simulink model "RC_top_ACU"  (R2018b)
settings: Solver=VariableStepAuto  StartTime=0.0  StopTime=500000.0  RelTol=1e-3
libraries: simulink x4
(part 2 of 3)

== system RC_top_ACU/Global Model RC/ACU/C_steam_4 ==
  from_T_prev_point : Inport
  from_T_curr_point : Inport  Port=2
  init_condition_curr_point : Inport  Port=3
  EVAP_params : Inport  Port=4
  from_prev_point : Inport  Port=5
  from_liquid : Inport  Port=6
  C_steam : Integrator  InitialConditionSource=external  InitialCondition=156.9966
  Gain29 : Gain  Gain=0.0000216487318*10^(-9)
  Sum3 : Sum  Inputs=-+-
  k1 : Subsystem
  speed : Subsystem
  to_next_point : Outport
  to_liquid : Outport  Port=2
  wires:
  init_condition_curr_point/1 -> C_steam/2
  speed/1(Out1) -> Sum3/2
  Gain29/1 -> Sum3/3
  Sum3/1 -> C_steam/1
  from_liquid/1 -> Gain29/1
  k1/1(Out1) -> Sum3/1
  C_steam/1 -> k1/2(In2), to_next_point/1, to_liquid/1
  from_T_curr_point/1 -> k1/1(In1)
  EVAP_params/1 -> k1/3(EVAP_params1), speed/3(EVAP_params)
  from_prev_point/1 -> speed/1(In1)
  from_T_prev_point/1 -> speed/2(In2)

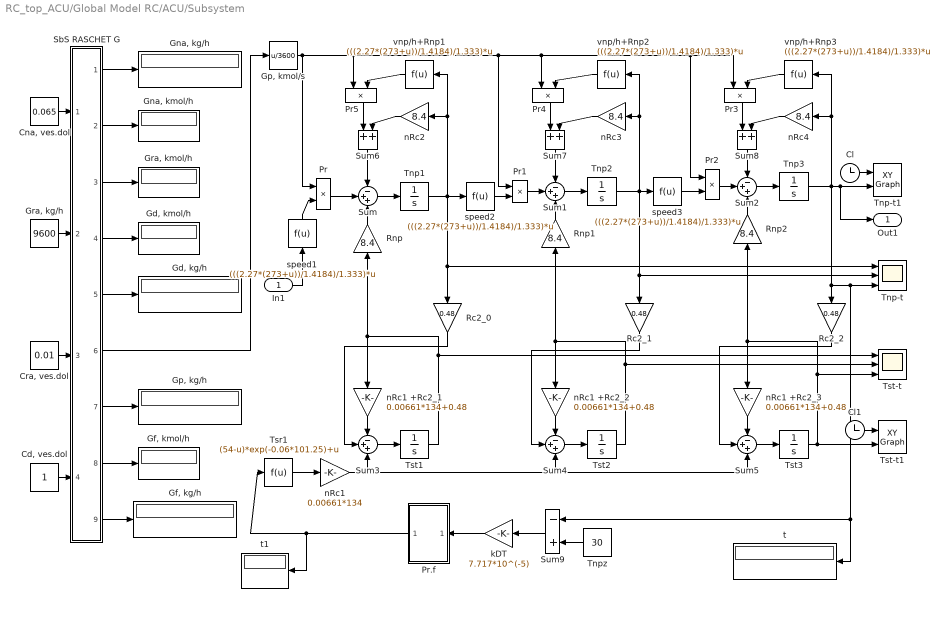
== system RC_top_ACU/Global Model RC/ACU/Subsystem ==
  In1 : Inport
  "Cd, ves.dol" : Constant
  Cl : Clock
  Cl1 : Clock
  "Cna, ves.dol" : Constant  Value=0.065
  "Cra, ves.dol" : Constant  Value=0.01
  "Gd, kg/h" : Display
  "Gd, kmol/h" : Display
  "Gf, kg/h" : Display
  "Gf, kmol/h" : Display
  "Gna, kg/h" : Display
  "Gna, kmol/h" : Display
  "Gp, kmol/s" : Fcn  Expr=u/3600
  "Gp, kg/h" : Display
  "Gra, kg/h" : Constant  Value=9600
  "Gra, kmol/h" : Display
  Pr{,1..5} (6 alike) : Product  RndMeth=Zero
  Pr.f : Subsystem
  Rc2_0 : Gain  Gain=0.48
  Rc2_1 : Gain  Gain=0.48
  Rc2_2 : Gain  Gain=0.48
  Rnp : Gain  Gain=8.4
  Rnp1 : Gain  Gain=8.4
  Rnp2 : Gain  Gain=8.4
  SbS RASCHET G : Subsystem
  Sum{,1..5} (6 alike) : Sum  Inputs=-++
  Sum6 : Sum
  Sum7 : Sum
  Sum8 : Sum
  Sum9 : Sum  Inputs=-+
  Tnp-t : Scope  NumInputPorts=3
  Tnp-t1 : simulink/Sinks/XY Graph  xmin=0  xmax=1000  ymin=10  ymax=50  st=-1
  Tnp1 : Integrator  InitialCondition=55.042986606641151
  Tnp2 : Integrator  InitialCondition=42.494060413287038
  Tnp3 : Integrator  InitialCondition=33.818616670435347
  Tnpz : Constant  Value=30
  Tsr1 : Fcn  Expr=(54-u)*exp(-0.06*101.25)+u
  Tst-t : Scope  NumInputPorts=3
  Tst-t1 : simulink/Sinks/XY Graph  xmin=0  xmax=1000  ymin=10  ymax=50  st=-1
  Tst1 : Integrator  InitialCondition=30.749212884999000
  Tst2 : Integrator  InitialCondition=26.338794670104530
  Tst3 : Integrator  InitialCondition=23.289742144317184
  kDT : Gain  Gain=7.717*10^(-5)
  nRc1 : Gain  Gain=0.00661*134
  nRc1 +Rc2_1 : Gain  Gain=0.00661*134+0.48
  nRc1 +Rc2_2 : Gain  Gain=0.00661*134+0.48
  nRc1 +Rc2_3 : Gain  Gain=0.00661*134+0.48
  nRc2 : Gain  Gain=8.4
  nRc3 : Gain  Gain=8.4
  nRc4 : Gain  Gain=8.4
  speed1 : Fcn  Expr=(((2.27*(273+u))/1.4184)/1.333)*u
  speed2 : Fcn  Expr=(((2.27*(273+u))/1.4184)/1.333)*u
  speed3 : Fcn  Expr=(((2.27*(273+u))/1.4184)/1.333)*u
  t : Display
  t1 : Display
  vnp/h+Rnp1 : Fcn  Expr=(((2.27*(273+u))/1.4184)/1.333)*u
  vnp/h+Rnp2 : Fcn  Expr=(((2.27*(273+u))/1.4184)/1.333)*u
  vnp/h+Rnp3 : Fcn  Expr=(((2.27*(273+u))/1.4184)/1.333)*u
  Out1 : Outport
  wires:
  Sum/1 -> Tnp1/1
  Tnp1/1 -> speed2/1, Rc2_0/1, Tnp-t/1, vnp/h+Rnp1/1, nRc2/1
  Sum1/1 -> Tnp2/1
  Tnp2/1 -> speed3/1, Rc2_1/1, Tnp-t/2, vnp/h+Rnp2/1, nRc3/1
  Sum2/1 -> Tnp3/1
  Tnp3/1 -> vnp/h+Rnp3/1, nRc4/1, Tnp-t1/2, Out1/1, Rc2_2/1, Tnp-t/3, t/1, Sum9/1
  Cl/1 -> Tnp-t1/1
  Rnp1/1 -> Sum1/3
  Rnp2/1 -> Sum2/3
  nRc1 +Rc2_1/1 -> Sum3/1
  Sum3/1 -> Tst1/1
  nRc1 +Rc2_2/1 -> Sum4/1
  Sum4/1 -> Tst2/1
  Tst2/1 -> nRc1 +Rc2_2/1, Rnp1/1, Tst-t/2
  nRc1 +Rc2_3/1 -> Sum5/1
  Sum5/1 -> Tst3/1
  nRc1/1 -> Sum3/3, Sum5/3, Sum4/3
  Rnp/1 -> Sum/3
  Tst1/1 -> nRc1 +Rc2_1/1, Rnp/1, Tst-t/1
  Tst3/1 -> Tst-t1/2, nRc1 +Rc2_3/1, Rnp2/1, Tst-t/3
  Rc2_1/1 -> Sum4/2
  Rc2_2/1 -> Sum5/2
  Rc2_0/1 -> Sum3/2
  Cl1/1 -> Tst-t1/1
  speed1/1 -> Pr/2
  "Gp, kmol/s"/1 -> Pr/1, Pr5/1, Pr2/1, Pr3/1, Pr4/1, Pr1/1
  Pr/1 -> Sum/2
  Pr1/1 -> Sum1/2
  speed2/1 -> Pr1/2
  Pr2/1 -> Sum2/2
  speed3/1 -> Pr2/2
  vnp/h+Rnp3/1 -> Pr3/2
  vnp/h+Rnp2/1 -> Pr4/2
  vnp/h+Rnp1/1 -> Pr5/2
  Pr5/1 -> Sum6/1
  Sum6/1 -> Sum/1
  nRc2/1 -> Sum6/2
  nRc3/1 -> Sum7/2
  Pr4/1 -> Sum7/1
  Sum7/1 -> Sum1/1
  nRc4/1 -> Sum8/2
  Pr3/1 -> Sum8/1
  Sum8/1 -> Sum2/1
  "Cna, ves.dol"/1 -> SbS RASCHET G/1(In1)
  "Cra, ves.dol"/1 -> SbS RASCHET G/3(In3)
  "Cd, ves.dol"/1 -> SbS RASCHET G/4(In4)
  "Gra, kg/h"/1 -> SbS RASCHET G/2(In2)
  SbS RASCHET G/1(Out1) -> "Gna, kg/h"/1
  SbS RASCHET G/5(Out5) -> "Gd, kg/h"/1
  SbS RASCHET G/7(Out7) -> "Gp, kg/h"/1
  SbS RASCHET G/9(Out9) -> "Gf, kg/h"/1
  SbS RASCHET G/2(Out2) -> "Gna, kmol/h"/1
  SbS RASCHET G/3(Out3) -> "Gra, kmol/h"/1
  SbS RASCHET G/4(Out4) -> "Gd, kmol/h"/1
  SbS RASCHET G/6(Out6) -> "Gp, kmol/s"/1
  SbS RASCHET G/8(Out8) -> "Gf, kmol/h"/1
  In1/1 -> speed1/1
  Sum9/1 -> kDT/1
  Tnpz/1 -> Sum9/2
  Pr.f/1(Out1) -> t1/1, Tsr1/1
  kDT/1 -> Pr.f/1(In1)
  Tsr1/1 -> nRc1/1

== system RC_top_ACU/Global Model RC/ACU/T_flue_1 ==
  init_condition_curr_point : Inport
  from_prev_point : Inport  Port=2
  from_side : Inport  Port=3
  Rdg : Gain  Gain=0.47
  Sum2 : Sum  Inputs=++-
  T_flue : Integrator  InitialConditionSource=external  InitialCondition=124.3766
  Vdg/h : Gain  Gain=4.6/1.375
  vdg/h+Rdg : Gain  Gain=4.6/1.375+0.47
  to_next_point : Outport
  to_side : Outport  Port=2
  wires:
  Vdg/h/1 -> Sum2/2
  from_prev_point/1 -> Vdg/h/1
  from_side/1 -> Rdg/1
  vdg/h+Rdg/1 -> Sum2/3
  Sum2/1 -> T_flue/1
  Rdg/1 -> Sum2/1
  init_condition_curr_point/1 -> T_flue/2
  T_flue/1 -> to_next_point/1, vdg/h+Rdg/1, to_side/1

== system RC_top_ACU/Global Model RC/ACU/T_flue_2 ==
  init_condition_curr_point : Inport
  from_prev_point : Inport  Port=2
  from_side : Inport  Port=3
  Rdg : Gain  Gain=0.47
  Sum2 : Sum  Inputs=++-
  T_flue : Integrator  InitialConditionSource=external  InitialCondition=124.3766
  Vdg/h : Gain  Gain=4.6/1.375
  vdg/h+Rdg : Gain  Gain=4.6/1.375+0.47
  to_next_point : Outport
  to_side : Outport  Port=2
  wires:
  Vdg/h/1 -> Sum2/2
  from_prev_point/1 -> Vdg/h/1
  from_side/1 -> Rdg/1
  vdg/h+Rdg/1 -> Sum2/3
  Sum2/1 -> T_flue/1
  Rdg/1 -> Sum2/1
  init_condition_curr_point/1 -> T_flue/2
  T_flue/1 -> to_next_point/1, vdg/h+Rdg/1, to_side/1

== system RC_top_ACU/Global Model RC/ACU/T_flue_3 ==
  init_condition_curr_point : Inport
  from_prev_point : Inport  Port=2
  from_side : Inport  Port=3
  Rdg : Gain  Gain=0.47
  Sum2 : Sum  Inputs=++-
  T_flue : Integrator  InitialConditionSource=external  InitialCondition=124.3766
  Vdg/h : Gain  Gain=4.6/1.375
  vdg/h+Rdg : Gain  Gain=4.6/1.375+0.47
  to_next_point : Outport
  to_side : Outport  Port=2
  wires:
  Vdg/h/1 -> Sum2/2
  from_prev_point/1 -> Vdg/h/1
  from_side/1 -> Rdg/1
  vdg/h+Rdg/1 -> Sum2/3
  Sum2/1 -> T_flue/1
  Rdg/1 -> Sum2/1
  init_condition_curr_point/1 -> T_flue/2
  T_flue/1 -> to_next_point/1, vdg/h+Rdg/1, to_side/1

== system RC_top_ACU/Global Model RC/ACU/T_flue_4 ==
  init_condition_curr_point : Inport
  from_prev_point : Inport  Port=2
  from_side : Inport  Port=3
  Rdg : Gain  Gain=0.47
  Sum2 : Sum  Inputs=++-
  T_flue : Integrator  InitialConditionSource=external  InitialCondition=124.3766
  Vdg/h : Gain  Gain=4.6/1.375
  vdg/h+Rdg : Gain  Gain=4.6/1.375+0.47
  to_next_point : Outport
  to_side : Outport  Port=2
  wires:
  Vdg/h/1 -> Sum2/2
  from_prev_point/1 -> Vdg/h/1
  from_side/1 -> Rdg/1
  vdg/h+Rdg/1 -> Sum2/3
  Sum2/1 -> T_flue/1
  Rdg/1 -> Sum2/1
  init_condition_curr_point/1 -> T_flue/2
  T_flue/1 -> to_next_point/1, vdg/h+Rdg/1, to_side/1

== system RC_top_ACU/Global Model RC/ACU/T_liquide_1 ==
  from_side : Inport
  init_condition_curr_point : Inport  Port=2
  from_prev_point : Inport  Port=3
  Ra : Gain  Gain=0.003
  Sum37 : Sum  Inputs=++-
  T_liquide : Integrator  InitialConditionSource=external  InitialCondition=136.285
  va/h+Ra : Gain  Gain=0.003/1.375+0.003
  va/h1 : Gain  Gain=0.003/1.375
  to_side : Outport
  to_next_point : Outport  Port=2
  wires:
  init_condition_curr_point/1 -> T_liquide/2
  va/h1/1 -> Sum37/2
  Sum37/1 -> T_liquide/1
  from_prev_point/1 -> va/h1/1
  Ra/1 -> Sum37/1
  from_side/1 -> Ra/1
  T_liquide/1 -> to_next_point/1, va/h+Ra/1, to_side/1
  va/h+Ra/1 -> Sum37/3

== system RC_top_ACU/Global Model RC/ACU/T_liquide_2 ==
  from_side : Inport
  init_condition_curr_point : Inport  Port=2
  from_prev_point : Inport  Port=3
  Ra : Gain  Gain=0.003
  Sum37 : Sum  Inputs=++-
  T_liquide : Integrator  InitialConditionSource=external  InitialCondition=136.285
  va/h+Ra : Gain  Gain=0.003/1.375+0.003
  va/h1 : Gain  Gain=0.003/1.375
  to_side : Outport
  to_next_point : Outport  Port=2
  wires:
  init_condition_curr_point/1 -> T_liquide/2
  va/h1/1 -> Sum37/2
  Sum37/1 -> T_liquide/1
  from_prev_point/1 -> va/h1/1
  Ra/1 -> Sum37/1
  from_side/1 -> Ra/1
  T_liquide/1 -> to_next_point/1, va/h+Ra/1, to_side/1
  va/h+Ra/1 -> Sum37/3

== system RC_top_ACU/Global Model RC/ACU/T_liquide_3 ==
  from_side : Inport
  init_condition_curr_point : Inport  Port=2
  from_prev_point : Inport  Port=3
  Ra : Gain  Gain=0.003
  Sum37 : Sum  Inputs=++-
  T_liquide : Integrator  InitialConditionSource=external  InitialCondition=136.285
  va/h+Ra : Gain  Gain=0.003/1.375+0.003
  va/h1 : Gain  Gain=0.003/1.375
  to_side : Outport
  to_next_point : Outport  Port=2
  wires:
  init_condition_curr_point/1 -> T_liquide/2
  va/h1/1 -> Sum37/2
  Sum37/1 -> T_liquide/1
  from_prev_point/1 -> va/h1/1
  Ra/1 -> Sum37/1
  from_side/1 -> Ra/1
  T_liquide/1 -> to_next_point/1, va/h+Ra/1, to_side/1
  va/h+Ra/1 -> Sum37/3

== system RC_top_ACU/Global Model RC/ACU/T_liquide_4 ==
  from_side : Inport
  init_condition_curr_point : Inport  Port=2
  from_prev_point : Inport  Port=3
  Ra : Gain  Gain=0.003
  Sum37 : Sum  Inputs=++-
  T_liquide : Integrator  InitialConditionSource=external  InitialCondition=136.285
  va/h+Ra : Gain  Gain=0.003/1.375+0.003
  va/h1 : Gain  Gain=0.003/1.375
  to_side : Outport
  to_next_point : Outport  Port=2
  wires:
  init_condition_curr_point/1 -> T_liquide/2
  va/h1/1 -> Sum37/2
  Sum37/1 -> T_liquide/1
  from_prev_point/1 -> va/h1/1
  Ra/1 -> Sum37/1
  from_side/1 -> Ra/1
  T_liquide/1 -> to_next_point/1, va/h+Ra/1, to_side/1
  va/h+Ra/1 -> Sum37/3

== system RC_top_ACU/Global Model RC/ACU/T_side_1 ==
  from_flue : Inport
  init_condition_curr_point : Inport  Port=2
  from_liquide : Inport  Port=3
  Rast : Gain  Gain=0.22
  Rdgst : Gain  Gain=0.008
  Rdgst+Rast : Gain  Gain=0.008+0.22
  Sum2 : Sum  Inputs=++-
  T_side : Integrator  InitialConditionSource=external  InitialCondition=124.3766
  to_flue : Outport
  to_liquide : Outport  Port=2
  wires:
  Rast/1 -> Sum2/2
  from_liquide/1 -> Rast/1
  from_flue/1 -> Rdgst/1
  T_side/1 -> Rdgst+Rast/1, to_liquide/1, to_flue/1
  Rdgst+Rast/1 -> Sum2/3
  Sum2/1 -> T_side/1
  Rdgst/1 -> Sum2/1
  init_condition_curr_point/1 -> T_side/2

== system RC_top_ACU/Global Model RC/ACU/T_side_2 ==
  from_flue : Inport
  init_condition_curr_point : Inport  Port=2
  from_liquide : Inport  Port=3
  Rast : Gain  Gain=0.22
  Rdgst : Gain  Gain=0.008
  Rdgst+Rast : Gain  Gain=0.008+0.22
  Sum2 : Sum  Inputs=++-
  T_side : Integrator  InitialConditionSource=external  InitialCondition=124.3766
  to_flue : Outport
  to_liquide : Outport  Port=2
  wires:
  Rast/1 -> Sum2/2
  from_liquide/1 -> Rast/1
  from_flue/1 -> Rdgst/1
  T_side/1 -> Rdgst+Rast/1, to_liquide/1, to_flue/1
  Rdgst+Rast/1 -> Sum2/3
  Sum2/1 -> T_side/1
  Rdgst/1 -> Sum2/1
  init_condition_curr_point/1 -> T_side/2

== system RC_top_ACU/Global Model RC/ACU/T_side_3 ==
  from_flue : Inport
  init_condition_curr_point : Inport  Port=2
  from_liquide : Inport  Port=3
  Rast : Gain  Gain=0.22
  Rdgst : Gain  Gain=0.008
  Rdgst+Rast : Gain  Gain=0.008+0.22
  Sum2 : Sum  Inputs=++-
  T_side : Integrator  InitialConditionSource=external  InitialCondition=124.3766
  to_flue : Outport
  to_liquide : Outport  Port=2
  wires:
  Rast/1 -> Sum2/2
  from_liquide/1 -> Rast/1
  from_flue/1 -> Rdgst/1
  T_side/1 -> Rdgst+Rast/1, to_liquide/1, to_flue/1
  Rdgst+Rast/1 -> Sum2/3
  Sum2/1 -> T_side/1
  Rdgst/1 -> Sum2/1
  init_condition_curr_point/1 -> T_side/2

== system RC_top_ACU/Global Model RC/ACU/T_side_4 ==
  from_flue : Inport
  init_condition_curr_point : Inport  Port=2
  from_liquide : Inport  Port=3
  Rast : Gain  Gain=0.22
  Rdgst : Gain  Gain=0.008
  Rdgst+Rast : Gain  Gain=0.008+0.22
  Sum2 : Sum  Inputs=++-
  T_side : Integrator  InitialConditionSource=external  InitialCondition=124.3766
  to_flue : Outport
  to_liquide : Outport  Port=2
  wires:
  Rast/1 -> Sum2/2
  from_liquide/1 -> Rast/1
  from_flue/1 -> Rdgst/1
  T_side/1 -> Rdgst+Rast/1, to_liquide/1, to_flue/1
  Rdgst+Rast/1 -> Sum2/3
  Sum2/1 -> T_side/1
  Rdgst/1 -> Sum2/1
  init_condition_curr_point/1 -> T_side/2

== system RC_top_ACU/Global Model RC/ACU/T_steam ==
  point_1 : Inport
  point_3 : Inport  Port=2
  point_2 : Inport  Port=3
  point_4 : Inport  Port=4
  Gain : Gain  Gain=1/4
  Sum37 : Sum  Inputs=++++
  to_side : Outport
  wires:
  point_2/1 -> Sum37/2
  point_1/1 -> Sum37/1
  point_3/1 -> Sum37/3
  point_4/1 -> Sum37/4
  Sum37/1 -> Gain/1
  Gain/1 -> to_side/1

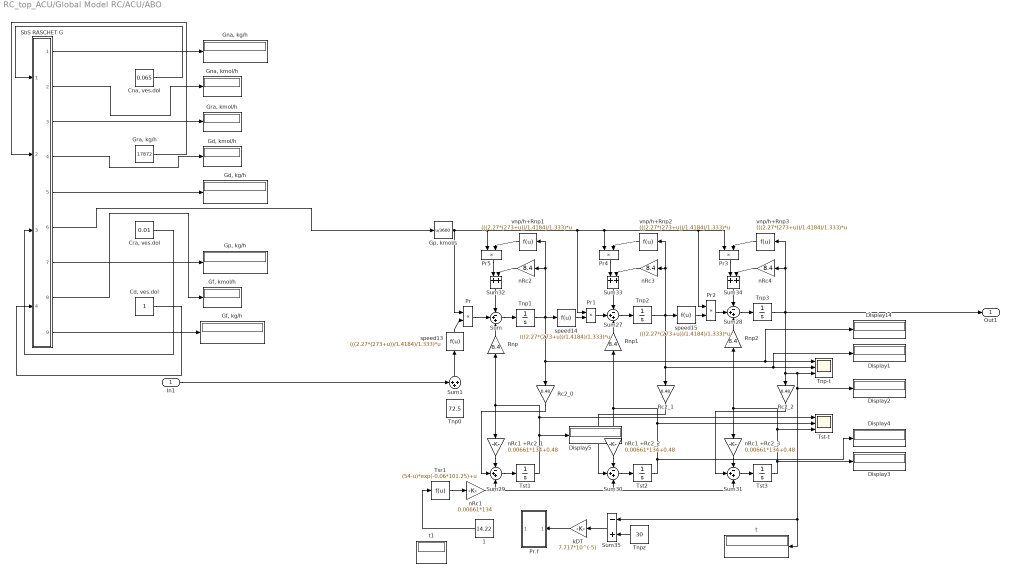
== system RC_top_ACU/Global Model RC/ACU/АВО ==
  In1 : Inport
  1 : Constant  Value=14.22
  "Cd, ves.dol" : Constant
  "Cna, ves.dol" : Constant  Value=0.065
  "Cra, ves.dol" : Constant  Value=0.01
  Display{1..5,14} (6 alike) : Display
  "Gd, kg/h" : Display
  "Gd, kmol/h" : Display
  "Gf, kg/h" : Display
  "Gf, kmol/h" : Display
  "Gna, kg/h" : Display
  "Gna, kmol/h" : Display
  "Gp, kmol/s" : Fcn  Expr=u/3600
  "Gp, kg/h" : Display
  "Gra, kg/h" : Constant  Value=17872
  "Gra, kmol/h" : Display
  Pr{,1..5} (6 alike) : Product  RndMeth=Zero
  Pr.f : Subsystem
  Rc2_0 : Gain  Gain=0.48
  Rc2_1 : Gain  Gain=0.48
  Rc2_2 : Gain  Gain=0.48
  Rnp : Gain  Gain=8.4
  Rnp1 : Gain  Gain=8.4
  Rnp2 : Gain  Gain=8.4
  SbS RASCHET G : Subsystem
  Sum{,27..31} (6 alike) : Sum  Inputs=-++
  Sum1 : Sum  Inputs=+++
  Sum32 : Sum
  Sum33 : Sum
  Sum34 : Sum
  Sum35 : Sum  Inputs=-+
  Tnp-t : Scope  NumInputPorts=3
  Tnp0 : Constant  Value=72.5
  Tnp1 : Integrator  InitialCondition=64.9985
  Tnp2 : Integrator  InitialCondition=57.497
  Tnp3 : Integrator  InitialCondition=49.9955
  Tnpz : Constant  Value=30
  Tsr1 : Fcn  Expr=(54-u)*exp(-0.06*101.25)+u
  Tst-t : Scope  NumInputPorts=3
  Tst1 : Integrator  InitialCondition=30.75
  Tst2 : Integrator  InitialCondition=27.02
  Tst3 : Integrator  InitialCondition=23.29
  kDT : Gain  Gain=7.717*10^(-5)
  nRc1 : Gain  Gain=0.00661*134
  nRc1 +Rc2_1 : Gain  Gain=0.00661*134+0.48
  nRc1 +Rc2_2 : Gain  Gain=0.00661*134+0.48
  nRc1 +Rc2_3 : Gain  Gain=0.00661*134+0.48
  nRc2 : Gain  Gain=8.4
  nRc3 : Gain  Gain=8.4
  nRc4 : Gain  Gain=8.4
  speed13 : Fcn  Expr=(((2.27*(273+u))/1.4184)/1.333)*u
  speed14 : Fcn  Expr=(((2.27*(273+u))/1.4184)/1.333)*u
  speed15 : Fcn  Expr=(((2.27*(273+u))/1.4184)/1.333)*u
  t : Display
  t1 : Display
  vnp/h+Rnp1 : Fcn  Expr=(((2.27*(273+u))/1.4184)/1.333)*u
  vnp/h+Rnp2 : Fcn  Expr=(((2.27*(273+u))/1.4184)/1.333)*u
  vnp/h+Rnp3 : Fcn  Expr=(((2.27*(273+u))/1.4184)/1.333)*u
  Out1 : Outport
  wires:
  Sum/1 -> Tnp1/1
  Tnp2/1 -> speed15/1, Rc2_1/1, Display1/1, Tnp-t/2, vnp/h+Rnp2/1, nRc3/1
  Tnp1/1 -> speed14/1, Rc2_0/1, Display14/1, Tnp-t/1, vnp/h+Rnp1/1, nRc2/1
  Sum27/1 -> Tnp2/1
  Sum28/1 -> Tnp3/1
  vnp/h+Rnp3/1 -> Pr3/2
  vnp/h+Rnp2/1 -> Pr4/2
  vnp/h+Rnp1/1 -> Pr5/2
  Sum32/1 -> Sum/1
  Rnp2/1 -> Sum28/3
  Pr4/1 -> Sum33/1
  "Cra, ves.dol"/1 -> SbS RASCHET G/3(In3)
  Sum31/1 -> Tst3/1
  "Cd, ves.dol"/1 -> SbS RASCHET G/4(In4)
  nRc1 +Rc2_1/1 -> Sum29/1
  Tst1/1 -> Display5/1, nRc1 +Rc2_1/1, Rnp/1, Tst-t/1
  "Gra, kg/h"/1 -> SbS RASCHET G/2(In2)
  SbS RASCHET G/1(Out1) -> "Gna, kg/h"/1
  SbS RASCHET G/5(Out5) -> "Gd, kg/h"/1
  Sum29/1 -> Tst1/1
  Pr/1 -> Sum/2
  Rc2_2/1 -> Sum31/2
  speed14/1 -> Pr1/2
  Rnp/1 -> Sum/3
  nRc1/1 -> Sum29/3, Sum31/3, Sum30/3
  "Gp, kmol/s"/1 -> Pr/1, Pr5/1, Pr2/1, Pr3/1, Pr4/1, Pr1/1
  Tnp3/1 -> vnp/h+Rnp3/1, nRc4/1, Out1/1, Rc2_2/1, Tnp-t/3, Display2/1, t/1, Sum35/1
  Tst3/1 -> Display3/1, nRc1 +Rc2_3/1, Rnp2/1, Tst-t/3
  Sum30/1 -> Tst2/1
  Pr5/1 -> Sum32/1
  Rc2_1/1 -> Sum30/2
  nRc1 +Rc2_3/1 -> Sum31/1
  Pr2/1 -> Sum28/2
  nRc2/1 -> Sum32/2
  nRc3/1 -> Sum33/2
  "Cna, ves.dol"/1 -> SbS RASCHET G/1(In1)
  speed15/1 -> Pr2/2
  Sum33/1 -> Sum27/1
  nRc4/1 -> Sum34/2
  Sum34/1 -> Sum28/1
  nRc1 +Rc2_2/1 -> Sum30/1
  Rnp1/1 -> Sum27/3
  Pr1/1 -> Sum27/2
  Pr3/1 -> Sum34/1
  speed13/1 -> Pr/2
  Tst2/1 -> nRc1 +Rc2_2/1, Rnp1/1, Tst-t/2, Display4/1
  Rc2_0/1 -> Sum29/2
  SbS RASCHET G/7(Out7) -> "Gp, kg/h"/1
  SbS RASCHET G/6(Out6) -> "Gp, kmol/s"/1
  SbS RASCHET G/4(Out4) -> "Gd, kmol/h"/1
  Tsr1/1 -> nRc1/1
  SbS RASCHET G/2(Out2) -> "Gna, kmol/h"/1
  SbS RASCHET G/3(Out3) -> "Gra, kmol/h"/1
  SbS RASCHET G/9(Out9) -> "Gf, kg/h"/1
  Sum35/1 -> kDT/1
  Tnpz/1 -> Sum35/2
  kDT/1 -> Pr.f/1(In1)
  SbS RASCHET G/8(Out8) -> "Gf, kmol/h"/1
  Sum1/1 -> speed13/1
  In1/1 -> Sum1/1
  1/1 -> Tsr1/1

== system RC_top_ACU/Global Model RC/FULL_RC_1/k19 ==
  In1 : Inport
  In2 : Inport  Port=2
  Product13 : Product  SaturateOnIntegerOverflow=on  InputSameDT=on  OutDataTypeStr=Inherit: Same as first input
  speed3 : Fcn  Expr=(0.002702752*(273.15+u))/1.17-0.147
  Out1 : Outport
  wires:
  Product13/1 -> Out1/1
  speed3/1 -> Product13/2
  In2/1 -> speed3/1
  In1/1 -> Product13/1

== system RC_top_ACU/Global Model RC/FULL_RC_1/k23 ==
  In1 : Inport
  In2 : Inport  Port=2
  Product13 : Product  SaturateOnIntegerOverflow=on  InputSameDT=on  OutDataTypeStr=Inherit: Same as first input
  speed3 : Fcn  Expr=(0.002702752*(273.15+u))/1.17-0.147
  Out1 : Outport
  wires:
  In1/1 -> Product13/1
  In2/1 -> speed3/1
  speed3/1 -> Product13/2
  Product13/1 -> Out1/1

== system RC_top_ACU/Global Model RC/FULL_RC_1/k24 ==
  In1 : Inport
  In2 : Inport  Port=2
  Product13 : Product  SaturateOnIntegerOverflow=on  InputSameDT=on  OutDataTypeStr=Inherit: Same as first input
  speed3 : Fcn  Expr=(0.002702752*(273.15+u))/1.17-0.147
  Out1 : Outport
  wires:
  Product13/1 -> Out1/1
  speed3/1 -> Product13/2
  In2/1 -> speed3/1
  In1/1 -> Product13/1

== system RC_top_ACU/Global Model RC/FULL_RC_1/k28 ==
  In1 : Inport
  In2 : Inport  Port=2
  Product13 : Product  SaturateOnIntegerOverflow=on  InputSameDT=on  OutDataTypeStr=Inherit: Same as first input
  speed3 : Fcn  Expr=((0.003223135*(273+u))/24.69822264)/0.5-0.004302
  Out1 : Outport
  wires:
  Product13/1 -> Out1/1
  speed3/1 -> Product13/1
  In1/1 -> speed3/1
  In2/1 -> Product13/2

== system RC_top_ACU/Global Model RC/FULL_RC_1/k29 ==
  In1 : Inport
  In2 : Inport  Port=2
  Product13 : Product  SaturateOnIntegerOverflow=on  InputSameDT=on  OutDataTypeStr=Inherit: Same as first input
  speed3 : Fcn  Expr=((0.003223135*(273+u))/24.69822264)/0.5-0.004302
  Out1 : Outport
  wires:
  Product13/1 -> Out1/1
  speed3/1 -> Product13/1
  In1/1 -> speed3/1
  In2/1 -> Product13/2

== system RC_top_ACU/Global Model RC/FULL_RC_1/k30 ==
  In1 : Inport
  In2 : Inport  Port=2
  Product13 : Product  SaturateOnIntegerOverflow=on  InputSameDT=on  OutDataTypeStr=Inherit: Same as first input
  speed3 : Fcn  Expr=((0.003223135*(273+u))/24.69822264)/0.5-0.004302
  Out1 : Outport
  wires:
  Product13/1 -> Out1/1
  speed3/1 -> Product13/1
  In1/1 -> speed3/1
  In2/1 -> Product13/2

== system RC_top_ACU/Global Model RC/FULL_RC_1/speed22 ==
  In1 : Inport
  In2 : Inport  Port=2
  Product13 : Product  SaturateOnIntegerOverflow=on  InputSameDT=on  OutDataTypeStr=Inherit: Same as first input
  speed3 : Fcn  Expr=(0.002702752*(273.15+u))/1.17
  Out1 : Outport
  wires:
  Product13/1 -> Out1/1
  speed3/1 -> Product13/2
  In2/1 -> speed3/1
  In1/1 -> Product13/1

== system RC_top_ACU/Global Model RC/FULL_RC_1/speed25 ==
  In1 : Inport
  In2 : Inport  Port=2
  Product13 : Product  SaturateOnIntegerOverflow=on  InputSameDT=on  OutDataTypeStr=Inherit: Same as first input
  speed3 : Fcn  Expr=((0.003223135*(273+u))/24.69822264)/0.5
  Out1 : Outport
  wires:
  In1/1 -> Product13/1
  In2/1 -> speed3/1
  speed3/1 -> Product13/2
  Product13/1 -> Out1/1

== system RC_top_ACU/Global Model RC/FULL_RC_1/speed26 ==
  In1 : Inport
  In2 : Inport  Port=2
  Product13 : Product  SaturateOnIntegerOverflow=on  InputSameDT=on  OutDataTypeStr=Inherit: Same as first input
  speed3 : Fcn  Expr=(0.002702752*(273.15+u))/1.17
  Out1 : Outport
  wires:
  In1/1 -> Product13/1
  In2/1 -> speed3/1
  speed3/1 -> Product13/2
  Product13/1 -> Out1/1

== system RC_top_ACU/Global Model RC/FULL_RC_1/speed30 ==
  In1 : Inport
  In2 : Inport  Port=2
  Product13 : Product  SaturateOnIntegerOverflow=on  InputSameDT=on  OutDataTypeStr=Inherit: Same as first input
  speed3 : Fcn  Expr=(0.002702752*(273.15+u))/1.17
  Out1 : Outport
  wires:
  In1/1 -> Product13/1
  In2/1 -> speed3/1
  speed3/1 -> Product13/2
  Product13/1 -> Out1/1

== system RC_top_ACU/Global Model RC/FULL_RC_1/speed31 ==
  In1 : Inport
  In2 : Inport  Port=2
  Product13 : Product  SaturateOnIntegerOverflow=on  InputSameDT=on  OutDataTypeStr=Inherit: Same as first input
  speed3 : Fcn  Expr=((0.003223135*(273+u))/24.69822264)/0.5
  Out1 : Outport
  wires:
  Product13/1 -> Out1/1
  In2/1 -> Product13/2
  speed3/1 -> Product13/1
  In1/1 -> speed3/1

== system RC_top_ACU/Global Model RC/FULL_RC_1/speed32 ==
  In1 : Inport
  In2 : Inport  Port=2
  Product13 : Product  SaturateOnIntegerOverflow=on  InputSameDT=on  OutDataTypeStr=Inherit: Same as first input
  speed3 : Fcn  Expr=((0.003223135*(273+u))/24.69822264)/0.5
  Out1 : Outport
  wires:
  Product13/1 -> Out1/1
  In2/1 -> Product13/2
  speed3/1 -> Product13/1
  In1/1 -> speed3/1

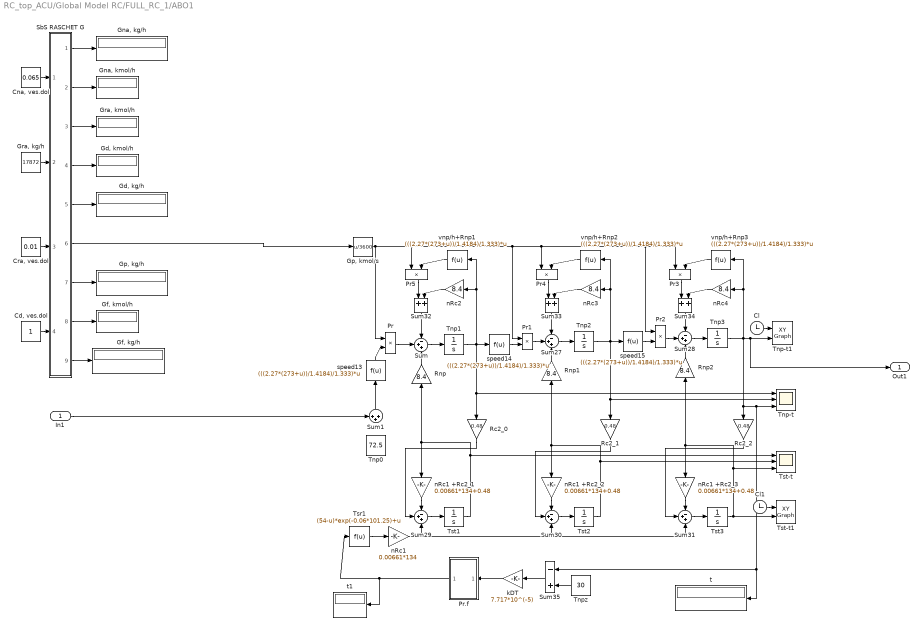
== system RC_top_ACU/Global Model RC/FULL_RC_1/АВО1 ==
  In1 : Inport
  "Cd, ves.dol" : Constant
  Cl : Clock
  Cl1 : Clock
  "Cna, ves.dol" : Constant  Value=0.065
  "Cra, ves.dol" : Constant  Value=0.01
  "Gd, kg/h" : Display
  "Gd, kmol/h" : Display
  "Gf, kg/h" : Display
  "Gf, kmol/h" : Display
  "Gna, kg/h" : Display
  "Gna, kmol/h" : Display
  "Gp, kmol/s" : Fcn  Expr=u/3600
  "Gp, kg/h" : Display
  "Gra, kg/h" : Constant  Value=17872
  "Gra, kmol/h" : Display
  Pr{,1..5} (6 alike) : Product  RndMeth=Zero
  Pr.f : Subsystem
  Rc2_0 : Gain  Gain=0.48
  Rc2_1 : Gain  Gain=0.48
  Rc2_2 : Gain  Gain=0.48
  Rnp : Gain  Gain=8.4
  Rnp1 : Gain  Gain=8.4
  Rnp2 : Gain  Gain=8.4
  SbS RASCHET G : Subsystem
  Sum{,27..31} (6 alike) : Sum  Inputs=-++
  Sum1 : Sum  Inputs=+++
  Sum32 : Sum
  Sum33 : Sum
  Sum34 : Sum
  Sum35 : Sum  Inputs=-+
  Tnp-t : Scope  NumInputPorts=3
  Tnp-t1 : simulink/Sinks/XY Graph  xmin=0  xmax=1000  ymin=10  ymax=50  st=-1
  Tnp0 : Constant  Value=72.5
  Tnp1 : Integrator  InitialCondition=55.042986606641151
  Tnp2 : Integrator  InitialCondition=42.494060413287038
  Tnp3 : Integrator  InitialCondition=33.818616670435347
  Tnpz : Constant  Value=30
  Tsr1 : Fcn  Expr=(54-u)*exp(-0.06*101.25)+u
  Tst-t : Scope  NumInputPorts=3
  Tst-t1 : simulink/Sinks/XY Graph  xmin=0  xmax=1000  ymin=10  ymax=50  st=-1
  Tst1 : Integrator  InitialCondition=30.749212884999000
  Tst2 : Integrator  InitialCondition=26.338794670104530
  Tst3 : Integrator  InitialCondition=23.289742144317184
  kDT : Gain  Gain=7.717*10^(-5)
  nRc1 : Gain  Gain=0.00661*134
  nRc1 +Rc2_1 : Gain  Gain=0.00661*134+0.48
  nRc1 +Rc2_2 : Gain  Gain=0.00661*134+0.48
  nRc1 +Rc2_3 : Gain  Gain=0.00661*134+0.48
  nRc2 : Gain  Gain=8.4
  nRc3 : Gain  Gain=8.4
  nRc4 : Gain  Gain=8.4
  speed13 : Fcn  Expr=(((2.27*(273+u))/1.4184)/1.333)*u
  speed14 : Fcn  Expr=(((2.27*(273+u))/1.4184)/1.333)*u
  speed15 : Fcn  Expr=(((2.27*(273+u))/1.4184)/1.333)*u
  t : Display
  t1 : Display
  vnp/h+Rnp1 : Fcn  Expr=(((2.27*(273+u))/1.4184)/1.333)*u
  vnp/h+Rnp2 : Fcn  Expr=(((2.27*(273+u))/1.4184)/1.333)*u
  vnp/h+Rnp3 : Fcn  Expr=(((2.27*(273+u))/1.4184)/1.333)*u
  Out1 : Outport
  wires:
  Sum/1 -> Tnp1/1
  Tnp2/1 -> speed15/1, Rc2_1/1, Tnp-t/2, vnp/h+Rnp2/1, nRc3/1
  Tnp1/1 -> speed14/1, Rc2_0/1, Tnp-t/1, vnp/h+Rnp1/1, nRc2/1
  Sum27/1 -> Tnp2/1
  Sum28/1 -> Tnp3/1
  vnp/h+Rnp3/1 -> Pr3/2
  vnp/h+Rnp2/1 -> Pr4/2
  vnp/h+Rnp1/1 -> Pr5/2
  Sum32/1 -> Sum/1
  Rnp2/1 -> Sum28/3
  Pr4/1 -> Sum33/1
  "Cra, ves.dol"/1 -> SbS RASCHET G/3(In3)
  Sum31/1 -> Tst3/1
  "Cd, ves.dol"/1 -> SbS RASCHET G/4(In4)
  Cl/1 -> Tnp-t1/1
  nRc1 +Rc2_1/1 -> Sum29/1
  Tst1/1 -> nRc1 +Rc2_1/1, Rnp/1, Tst-t/1
  "Gra, kg/h"/1 -> SbS RASCHET G/2(In2)
  SbS RASCHET G/1(Out1) -> "Gna, kg/h"/1
  SbS RASCHET G/5(Out5) -> "Gd, kg/h"/1
  Sum29/1 -> Tst1/1
  Pr/1 -> Sum/2
  Rc2_2/1 -> Sum31/2
  speed14/1 -> Pr1/2
  Rnp/1 -> Sum/3
  nRc1/1 -> Sum29/3, Sum31/3, Sum30/3
  "Gp, kmol/s"/1 -> Pr/1, Pr5/1, Pr2/1, Pr3/1, Pr4/1, Pr1/1
  Tnp3/1 -> vnp/h+Rnp3/1, nRc4/1, Out1/1, Tnp-t1/2, Rc2_2/1, Tnp-t/3, t/1, Sum35/1
  Tst3/1 -> Tst-t1/2, nRc1 +Rc2_3/1, Rnp2/1, Tst-t/3
  Sum30/1 -> Tst2/1
  Pr5/1 -> Sum32/1
  Rc2_1/1 -> Sum30/2
  nRc1 +Rc2_3/1 -> Sum31/1
  Pr2/1 -> Sum28/2
  nRc2/1 -> Sum32/2
  nRc3/1 -> Sum33/2
  "Cna, ves.dol"/1 -> SbS RASCHET G/1(In1)
  speed15/1 -> Pr2/2
  Sum33/1 -> Sum27/1
  nRc4/1 -> Sum34/2
  Sum34/1 -> Sum28/1
  nRc1 +Rc2_2/1 -> Sum30/1
  Rnp1/1 -> Sum27/3
  Cl1/1 -> Tst-t1/1
  Pr1/1 -> Sum27/2
  Pr3/1 -> Sum34/1
  speed13/1 -> Pr/2
  Tst2/1 -> nRc1 +Rc2_2/1, Rnp1/1, Tst-t/2
  Rc2_0/1 -> Sum29/2
  SbS RASCHET G/7(Out7) -> "Gp, kg/h"/1
  SbS RASCHET G/6(Out6) -> "Gp, kmol/s"/1
  SbS RASCHET G/4(Out4) -> "Gd, kmol/h"/1
  Tsr1/1 -> nRc1/1
  SbS RASCHET G/2(Out2) -> "Gna, kmol/h"/1
  SbS RASCHET G/3(Out3) -> "Gra, kmol/h"/1
  Pr.f/1(Out1) -> t1/1, Tsr1/1
  SbS RASCHET G/9(Out9) -> "Gf, kg/h"/1
  Sum35/1 -> kDT/1
  Tnpz/1 -> Sum35/2
  kDT/1 -> Pr.f/1(In1)
  SbS RASCHET G/8(Out8) -> "Gf, kmol/h"/1
  Sum1/1 -> speed13/1
  In1/1 -> Sum1/1

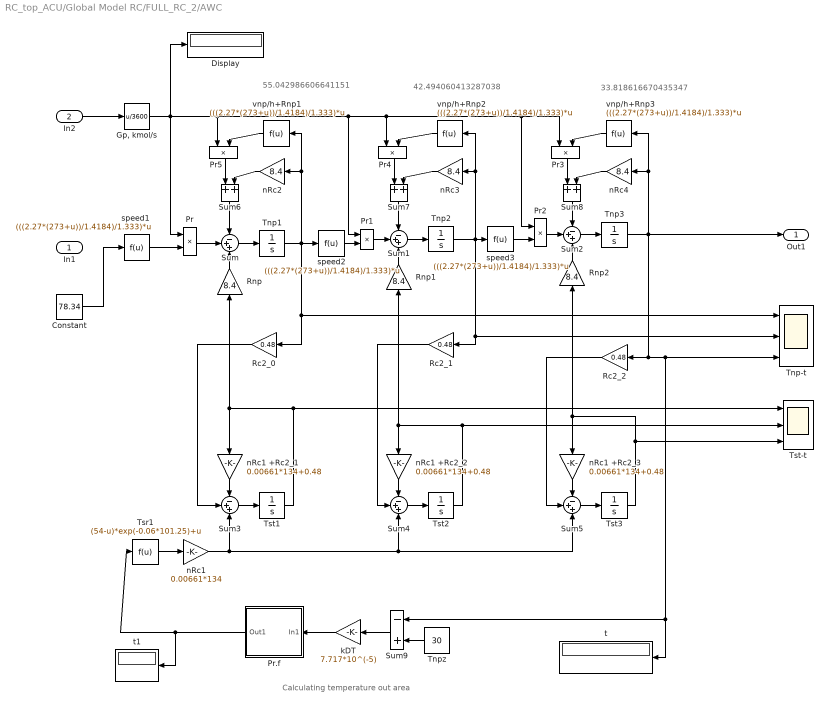
== system RC_top_ACU/Global Model RC/FULL_RC_2/AWC ==
  note: 33.818616670435347
  note: 42.494060413287038
  note: 55.042986606641151
  note: Calculating temperature out area
  In1 : Inport
  In2 : Inport  Port=2
  Constant : Constant  Value=78.34
  Display : Display
  "Gp, kmol/s" : Fcn  Expr=u/3600
  Pr{,1..5} (6 alike) : Product  RndMeth=Zero
  Pr.f : Subsystem
  Rc2_0 : Gain  Gain=0.48
  Rc2_1 : Gain  Gain=0.48
  Rc2_2 : Gain  Gain=0.48
  Rnp : Gain  Gain=8.4
  Rnp1 : Gain  Gain=8.4
  Rnp2 : Gain  Gain=8.4
  Sum{,1..5} (6 alike) : Sum  Inputs=-++
  Sum6 : Sum
  Sum7 : Sum
  Sum8 : Sum
  Sum9 : Sum  Inputs=-+
  Tnp-t : Scope  NumInputPorts=3
  Tnp1 : Integrator  InitialCondition=55.042986606641151
  Tnp2 : Integrator  InitialCondition=42.494060413287038
  Tnp3 : Integrator  InitialCondition=33.818616670435347
  Tnpz : Constant  Value=30
  Tsr1 : Fcn  Expr=(54-u)*exp(-0.06*101.25)+u
  Tst-t : Scope  NumInputPorts=3
  Tst1 : Integrator  InitialCondition=30.749212884999000
  Tst2 : Integrator  InitialCondition=26.338794670104530
  Tst3 : Integrator  InitialCondition=23.289742144317184
  kDT : Gain  Gain=7.717*10^(-5)
  nRc1 : Gain  Gain=0.00661*134
  nRc1 +Rc2_1 : Gain  Gain=0.00661*134+0.48
  nRc1 +Rc2_2 : Gain  Gain=0.00661*134+0.48
  nRc1 +Rc2_3 : Gain  Gain=0.00661*134+0.48
  nRc2 : Gain  Gain=8.4
  nRc3 : Gain  Gain=8.4
  nRc4 : Gain  Gain=8.4
  speed1 : Fcn  Expr=(((2.27*(273+u))/1.4184)/1.333)*u
  speed2 : Fcn  Expr=(((2.27*(273+u))/1.4184)/1.333)*u
  speed3 : Fcn  Expr=(((2.27*(273+u))/1.4184)/1.333)*u
  t : Display
  t1 : Display
  vnp/h+Rnp1 : Fcn  Expr=(((2.27*(273+u))/1.4184)/1.333)*u
  vnp/h+Rnp2 : Fcn  Expr=(((2.27*(273+u))/1.4184)/1.333)*u
  vnp/h+Rnp3 : Fcn  Expr=(((2.27*(273+u))/1.4184)/1.333)*u
  Out1 : Outport
  wires:
  Sum/1 -> Tnp1/1
  Tnp1/1 -> speed2/1, Rc2_0/1, Tnp-t/1, vnp/h+Rnp1/1, nRc2/1
  Sum1/1 -> Tnp2/1
  Tnp2/1 -> speed3/1, Rc2_1/1, Tnp-t/2, vnp/h+Rnp2/1, nRc3/1
  Sum2/1 -> Tnp3/1
  Tnp3/1 -> vnp/h+Rnp3/1, nRc4/1, Out1/1, Rc2_2/1, Tnp-t/3, t/1, Sum9/1
  Rnp1/1 -> Sum1/3
  Rnp2/1 -> Sum2/3
  nRc1 +Rc2_1/1 -> Sum3/1
  Sum3/1 -> Tst1/1
  nRc1 +Rc2_2/1 -> Sum4/1
  Sum4/1 -> Tst2/1
  Tst2/1 -> Rnp1/1, nRc1 +Rc2_2/1, Tst-t/2
  nRc1 +Rc2_3/1 -> Sum5/1
  Sum5/1 -> Tst3/1
  nRc1/1 -> Sum3/3, Sum4/3, Sum5/3
  Rnp/1 -> Sum/3
  Tst1/1 -> nRc1 +Rc2_1/1, Rnp/1, Tst-t/1
  Tst3/1 -> Rnp2/1, nRc1 +Rc2_3/1, Tst-t/3
  Rc2_1/1 -> Sum4/2
  Rc2_2/1 -> Sum5/2
  Rc2_0/1 -> Sum3/2
  speed1/1 -> Pr/2
  "Gp, kmol/s"/1 -> Display/1, Pr/1, Pr5/1, Pr2/1, Pr3/1, Pr4/1, Pr1/1
  Pr/1 -> Sum/2
  Pr1/1 -> Sum1/2
  speed2/1 -> Pr1/2
  Pr2/1 -> Sum2/2
  speed3/1 -> Pr2/2
  vnp/h+Rnp3/1 -> Pr3/2
  vnp/h+Rnp2/1 -> Pr4/2
  vnp/h+Rnp1/1 -> Pr5/2
  Pr5/1 -> Sum6/1
  Sum6/1 -> Sum/1
  nRc2/1 -> Sum6/2
  nRc3/1 -> Sum7/2
  Pr4/1 -> Sum7/1
  Sum7/1 -> Sum1/1
  nRc4/1 -> Sum8/2
  Pr3/1 -> Sum8/1
  Sum8/1 -> Sum2/1
  Sum9/1 -> kDT/1
  Tnpz/1 -> Sum9/2
  Pr.f/1(Out1) -> t1/1, Tsr1/1
  kDT/1 -> Pr.f/1(In1)
  Tsr1/1 -> nRc1/1
  In2/1 -> "Gp, kmol/s"/1
  Constant/1 -> speed1/1

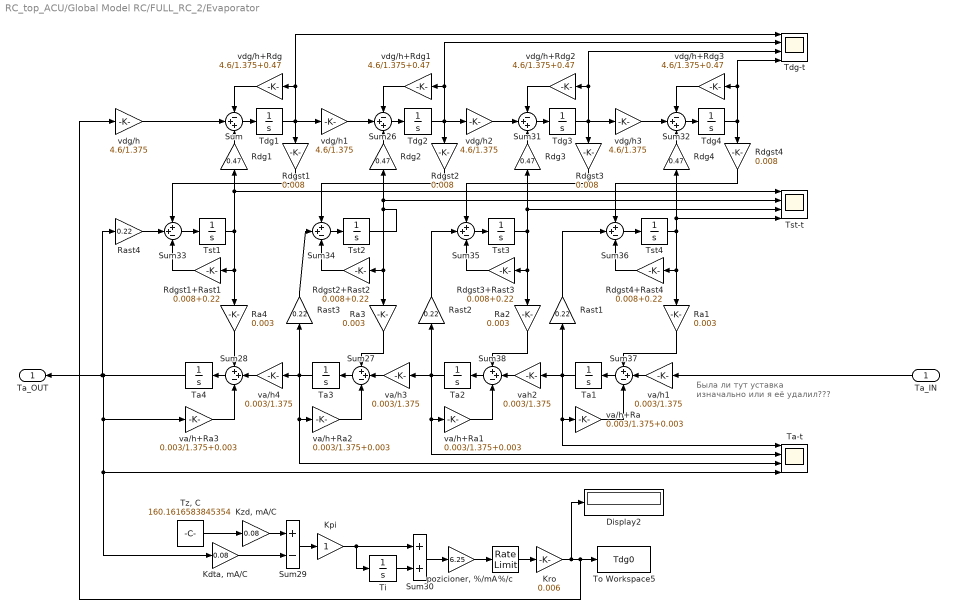
== system RC_top_ACU/Global Model RC/FULL_RC_2/Evaporator ==
  note: Была ли тут уставка изначально или я её удалил???
  Ta_IN : Inport
  %/c : RateLimiter  RisingSlewLimit=5  FallingSlewLimit=-5  SampleTimeMode=inherited
  Display2 : Display
  "Kdta, mA/C" : Gain  Gain=0.08
  Kpi : Gain
  Kro : Gain  Gain=0.006
  "Kzd, mA/C" : Gain  Gain=0.08
  Ra{1..4} (4 alike) : Gain  Gain=0.003
  Rast{1..4} (4 alike) : Gain  Gain=0.22
  Rdg{1..4} (4 alike) : Gain  Gain=0.47
  Rdgst{1..4} (4 alike) : Gain  Gain=0.008
  Rdgst1+Rast1 : Gain  Gain=0.008+0.22
  Rdgst2+Rast2 : Gain  Gain=0.008+0.22
  Rdgst3+Rast3 : Gain  Gain=0.008+0.22
  Rdgst4+Rast4 : Gain  Gain=0.008+0.22
  Sum{,26,31..32} (4 alike) : Sum  Inputs=-++
  Sum{27..28,33..38} (8 alike) : Sum  Inputs=++-
  Sum29 : Sum  Inputs=+-
  Sum30 : Sum
  Ta-t : Scope  NumInputPorts=4
  Ta1 : Integrator  InitialCondition=136.285
  Ta2 : Integrator  InitialCondition=144.19
  Ta3 : Integrator  InitialCondition=152.09
  Ta4 : Integrator  InitialCondition=160
  Tdg-t : Scope  NumInputPorts=4
  Tdg1 : Integrator  InitialCondition=283.3065209436467
  Tdg2 : Integrator  InitialCondition=267.8966165589237
  Tdg3 : Integrator  InitialCondition=253.6715917846216
  Tdg4 : Integrator  InitialCondition=240.5403403000344
  Ti : Integrator  InitialCondition=8000  UpperSaturationLimit=8012  LowerSaturationLimit=6012
  To Workspace5 : ToWorkspace  VariableName=Tdg0  SampleTime=-1
  Tst-t : Scope  NumInputPorts=4
  Tst1 : Integrator  InitialCondition=164.4825307550351
  Tst2 : Integrator  InitialCondition=158.2090959868120
  Tst3 : Integrator  InitialCondition=152.4180305285302
  Tst4 : Integrator  InitialCondition=147.0722446263660
  "Tz, C" : Constant  Value=160.1616583845354
  "pozicioner, %/mA" : Gain  Gain=6.25
  va/h+Ra{,1..3} (4 alike) : Gain  Gain=0.003/1.375+0.003
  va/h1 : Gain  Gain=0.003/1.375
  va/h3 : Gain  Gain=0.003/1.375
  va/h4 : Gain  Gain=0.003/1.375
  vah2 : Gain  Gain=0.003/1.375
  vdg/h{,1..3} (4 alike) : Gain  Gain=4.6/1.375
  vdg/h+Rdg{,1..3} (4 alike) : Gain  Gain=4.6/1.375+0.47
  Ta_OUT : Outport
  wires:
  Sum/1 -> Tdg1/1
  vdg/h2/1 -> Sum31/2
  Sum32/1 -> Tdg4/1
  Tdg2/1 -> vdg/h+Rdg1/1, Tdg-t/2, Rdgst2/1, vdg/h2/1
  Sum26/1 -> Tdg2/1
  vdg/h3/1 -> Sum32/2
  vdg/h/1 -> Sum/2
  Tdg1/1 -> vdg/h+Rdg/1, Tdg-t/1, vdg/h1/1, Rdgst1/1
  vdg/h+Rdg2/1 -> Sum31/1
  vdg/h+Rdg3/1 -> Sum32/1
  Tdg4/1 -> vdg/h+Rdg3/1, Tdg-t/4, Rdgst4/1
  Rdg1/1 -> Sum/3
  Rdg2/1 -> Sum26/3
  Rdg3/1 -> Sum31/3
  Rdg4/1 -> Sum32/3
  vdg/h+Rdg1/1 -> Sum26/1
  Sum33/1 -> Tst1/1
  Sum34/1 -> Tst2/1
  Tdg3/1 -> vdg/h+Rdg2/1, Tdg-t/3, vdg/h3/1, Rdgst3/1
  vdg/h1/1 -> Sum26/2
  Sum35/1 -> Tst3/1
  vdg/h+Rdg/1 -> Sum/1
  Sum31/1 -> Tdg3/1
  Rdgst3+Rast3/1 -> Sum35/3
  Tst1/1 -> Rdgst1+Rast1/1, Ra4/1, Rdg1/1, Tst-t/1
  Rdgst1+Rast1/1 -> Sum33/3
  Tst3/1 -> Rdgst3+Rast3/1, Ra2/1, Rdg3/1, Tst-t/3
  Tst2/1 -> Rdg2/1, Tst-t/2, Rdgst2+Rast2/1, Ra3/1
  Rdgst1/1 -> Sum33/1
  Rdgst2/1 -> Sum34/1
  Tst4/1 -> Rdgst4+Rast4/1, Ra1/1, Rdg4/1, Tst-t/4
  Rdgst4/1 -> Sum36/1
  Rdgst2+Rast2/1 -> Sum34/3
  va/h1/1 -> Sum37/2
  va/h+Ra/1 -> Sum37/3
  Rdgst3/1 -> Sum35/1
  Sum36/1 -> Tst4/1
  Rdgst4+Rast4/1 -> Sum36/3
  Ti/1 -> Sum30/2
  Ta4/1 -> Ta_OUT/1, Rast4/1, va/h+Ra3/1, Ta-t/4, "Kdta, mA/C"/1
  Rast1/1 -> Sum36/2
  Ra2/1 -> Sum38/1
  Ta2/1 -> va/h+Ra1/1, Ta-t/2, va/h3/1, Rast2/1
  va/h+Ra3/1 -> Sum28/3
  Ta1/1 -> Ta-t/1, va/h+Ra/1, Rast1/1, vah2/1
  va/h+Ra2/1 -> Sum27/3
  Rast3/1 -> Sum34/2
  Sum38/1 -> Ta2/1
  va/h4/1 -> Sum28/2
  Sum37/1 -> Ta1/1
  va/h3/1 -> Sum27/2
  Ta3/1 -> va/h+Ra2/1, Ta-t/3, va/h4/1, Rast3/1
  Rast2/1 -> Sum35/2
  "Tz, C"/1 -> "Kzd, mA/C"/1
  "Kdta, mA/C"/1 -> Sum29/2
  %/c/1 -> Kro/1
  Ta_IN/1 -> va/h1/1
  "Kzd, mA/C"/1 -> Sum29/1
  Sum28/1 -> Ta4/1
  Rast4/1 -> Sum33/2
  Sum27/1 -> Ta3/1
  va/h+Ra1/1 -> Sum38/3
  "pozicioner, %/mA"/1 -> %/c/1
  Ra3/1 -> Sum27/1
  Sum29/1 -> Kpi/1
  Kpi/1 -> Sum30/1, Ti/1
  Ra4/1 -> Sum28/1
  Sum30/1 -> "pozicioner, %/mA"/1
  Kro/1 -> To Workspace5/1, vdg/h/1, Display2/1
  Ra1/1 -> Sum37/1
  vah2/1 -> Sum38/2

== system RC_top_ACU/Global Model RC/FULL_RC_2/G() ==
  "Cd, ves.dol" : Constant
  "Cna, ves.dol" : Constant  Value=0.065
  "Cra, ves.dol" : Constant  Value=0.01
  "Gd, kg/h" : Display
  "Gd, kmol/h" : Display
  "Gf, kg/h" : Display
  "Gf, kmol/h" : Display
  "Gna, kg/h" : Display
  "Gna, kmol/h" : Display
  "Gp, kg/h" : Display
  "Gra, kg/h" : Constant  Value=9600
  "Gra, kmol/h" : Display
  SbS RASCHET G : Subsystem
  Out1 : Outport
  wires:
  SbS RASCHET G/2(Out2) -> "Gna, kmol/h"/1
  "Cra, ves.dol"/1 -> SbS RASCHET G/3(In3)
  "Cna, ves.dol"/1 -> SbS RASCHET G/1(In1)
  SbS RASCHET G/1(Out1) -> "Gna, kg/h"/1
  "Cd, ves.dol"/1 -> SbS RASCHET G/4(In4)
  "Gra, kg/h"/1 -> SbS RASCHET G/2(In2)
  SbS RASCHET G/7(Out7) -> "Gp, kg/h"/1
  SbS RASCHET G/9(Out9) -> "Gf, kg/h"/1
  SbS RASCHET G/8(Out8) -> "Gf, kmol/h"/1
  SbS RASCHET G/4(Out4) -> "Gd, kmol/h"/1
  SbS RASCHET G/5(Out5) -> "Gd, kg/h"/1
  SbS RASCHET G/3(Out3) -> "Gra, kmol/h"/1
  SbS RASCHET G/6(Out6) -> Out1/1

== system RC_top_ACU/Global Model RC/FULL_RC_2/k31 ==
  In1 : Inport
  In2 : Inport  Port=2
  Product13 : Product  SaturateOnIntegerOverflow=on  InputSameDT=on  OutDataTypeStr=Inherit: Same as first input
  speed3 : Fcn  Expr=((0.003223135*(273+u))/24.69822264)/0.5-0.0216487318
  Out1 : Outport
  wires:
  Product13/1 -> Out1/1
  speed3/1 -> Product13/1
  In1/1 -> speed3/1
  In2/1 -> Product13/2

== system RC_top_ACU/Global Model RC/FULL_RC_2/k32 ==
  In1 : Inport
  In2 : Inport  Port=2
  Product13 : Product  SaturateOnIntegerOverflow=on  InputSameDT=on  OutDataTypeStr=Inherit: Same as first input
  speed3 : Fcn  Expr=(0.002702752*(273.15+u))/1.17-0.147
  Out1 : Outport
  wires:
  Product13/1 -> Out1/1
  speed3/1 -> Product13/2
  In2/1 -> speed3/1
  In1/1 -> Product13/1

== system RC_top_ACU/Global Model RC/FULL_RC_2/k33 ==
  In1 : Inport
  In2 : Inport  Port=2
  Product13 : Product  SaturateOnIntegerOverflow=on  InputSameDT=on  OutDataTypeStr=Inherit: Same as first input
  speed3 : Fcn  Expr=(0.002702752*(273.15+u))/1.17-0.147
  Out1 : Outport
  wires:
  In1/1 -> Product13/1
  In2/1 -> speed3/1
  speed3/1 -> Product13/2
  Product13/1 -> Out1/1

== system RC_top_ACU/Global Model RC/FULL_RC_2/k34 ==
  In1 : Inport
  In2 : Inport  Port=2
  Product13 : Product  SaturateOnIntegerOverflow=on  InputSameDT=on  OutDataTypeStr=Inherit: Same as first input
  speed3 : Fcn  Expr=(0.002702752*(273.15+u))/1.17-0.147
  Out1 : Outport
  wires:
  Product13/1 -> Out1/1
  speed3/1 -> Product13/2
  In2/1 -> speed3/1
  In1/1 -> Product13/1

== system RC_top_ACU/Global Model RC/FULL_RC_2/k38 ==
  In1 : Inport
  In2 : Inport  Port=2
  Product13 : Product  SaturateOnIntegerOverflow=on  InputSameDT=on  OutDataTypeStr=Inherit: Same as first input
  speed3 : Fcn  Expr=((0.003223135*(273+u))/24.69822264)/0.5-0.0216487318
  Out1 : Outport
  wires:
  Product13/1 -> Out1/1
  speed3/1 -> Product13/1
  In1/1 -> speed3/1
  In2/1 -> Product13/2

== system RC_top_ACU/Global Model RC/FULL_RC_2/k39 ==
  In1 : Inport
  In2 : Inport  Port=2
  Product13 : Product  SaturateOnIntegerOverflow=on  InputSameDT=on  OutDataTypeStr=Inherit: Same as first input
  speed3 : Fcn  Expr=((0.003223135*(273+u))/24.69822264)/0.5-0.0216487318
  Out1 : Outport
  wires:
  Product13/1 -> Out1/1
  speed3/1 -> Product13/1
  In1/1 -> speed3/1
  In2/1 -> Product13/2

== system RC_top_ACU/Global Model RC/FULL_RC_2/speed34 ==
  In1 : Inport
  In2 : Inport  Port=2
  Product13 : Product  SaturateOnIntegerOverflow=on  InputSameDT=on  OutDataTypeStr=Inherit: Same as first input
  speed3 : Fcn  Expr=((0.003223135*(273+u))/24.69822264)/0.5
  Out1 : Outport
  wires:
  Product13/1 -> Out1/1
  In2/1 -> Product13/2
  speed3/1 -> Product13/1
  In1/1 -> speed3/1

== system RC_top_ACU/Global Model RC/FULL_RC_2/speed35 ==
  In1 : Inport
  In2 : Inport  Port=2
  Product13 : Product  SaturateOnIntegerOverflow=on  InputSameDT=on  OutDataTypeStr=Inherit: Same as first input
  speed3 : Fcn  Expr=(0.002702752*(273.15+u))/1.17
  Out1 : Outport
  wires:
  Product13/1 -> Out1/1
  speed3/1 -> Product13/2
  In2/1 -> speed3/1
  In1/1 -> Product13/1

== system RC_top_ACU/Global Model RC/FULL_RC_2/speed36 ==
  In1 : Inport
  In2 : Inport  Port=2
  Product13 : Product  SaturateOnIntegerOverflow=on  InputSameDT=on  OutDataTypeStr=Inherit: Same as first input
  speed3 : Fcn  Expr=(0.002702752*(273.15+u))/1.17
  Out1 : Outport
  wires:
  In1/1 -> Product13/1
  In2/1 -> speed3/1
  speed3/1 -> Product13/2
  Product13/1 -> Out1/1

== system RC_top_ACU/Global Model RC/FULL_RC_2/speed40 ==
  In1 : Inport
  In2 : Inport  Port=2
  Product13 : Product  SaturateOnIntegerOverflow=on  InputSameDT=on  OutDataTypeStr=Inherit: Same as first input
  speed3 : Fcn  Expr=(0.002702752*(273.15+u))/1.17
  Out1 : Outport
  wires:
  In1/1 -> Product13/1
  In2/1 -> speed3/1
  speed3/1 -> Product13/2
  Product13/1 -> Out1/1

== system RC_top_ACU/Global Model RC/FULL_RC_2/speed41 ==
  In1 : Inport
  In2 : Inport  Port=2
  Product13 : Product  SaturateOnIntegerOverflow=on  InputSameDT=on  OutDataTypeStr=Inherit: Same as first input
  speed3 : Fcn  Expr=((0.003223135*(273+u))/24.69822264)/0.5
  Out1 : Outport
  wires:
  Product13/1 -> Out1/1
  In2/1 -> Product13/2
  speed3/1 -> Product13/1
  In1/1 -> speed3/1

== system RC_top_ACU/Global Model RC/FULL_RC_2/speed45 ==
  In1 : Inport
  In2 : Inport  Port=2
  Product13 : Product  SaturateOnIntegerOverflow=on  InputSameDT=on  OutDataTypeStr=Inherit: Same as first input
  speed3 : Fcn  Expr=((0.003223135*(273+u))/24.69822264)/0.5
  Out1 : Outport
  wires:
  In1/1 -> Product13/1
  In2/1 -> speed3/1
  speed3/1 -> Product13/2
  Product13/1 -> Out1/1

== system RC_top_ACU/Global Model RC/RC_top/C_liquide_1 ==
  from_steam : Inport
  from_prev_point : Inport  Port=2
  init_condition_curr_point : Inport  Port=3
  Gain18 : Gain  Gain=0.000006
  Gain19 : Gain  Gain=0.00004/1.17
  Gain22 : Gain  Gain=0.00004/1.17-(0.000006*0.000000000145)
  Sum2 : Sum  Inputs=-+-
  Tl1 : Integrator  InitialConditionSource=external  InitialCondition=124.3766
  to_steam : Outport
  to_next_point : Outport  Port=2
  wires:
  Gain22/1 -> Sum2/3
  Gain19/1 -> Sum2/2
  Sum2/1 -> Tl1/1
  Tl1/1 -> Gain22/1, to_steam/1, to_next_point/1
  Gain18/1 -> Sum2/1
  init_condition_curr_point/1 -> Tl1/2
  from_prev_point/1 -> Gain19/1
  from_steam/1 -> Gain18/1

== system RC_top_ACU/Global Model RC/RC_top/C_liquide_2 ==
  from_steam : Inport
  from_prev_point : Inport  Port=2
  init_condition_curr_point : Inport  Port=3
  Gain18 : Gain  Gain=0.000006
  Gain19 : Gain  Gain=0.00004/1.17
  Gain22 : Gain  Gain=0.00004/1.17-(0.000006*0.000000000145)
  Sum2 : Sum  Inputs=-+-
  Tl1 : Integrator  InitialConditionSource=external  InitialCondition=124.3766
  to_steam : Outport
  to_next_point : Outport  Port=2
  wires:
  Gain22/1 -> Sum2/3
  Gain19/1 -> Sum2/2
  Sum2/1 -> Tl1/1
  Tl1/1 -> Gain22/1, to_steam/1, to_next_point/1
  Gain18/1 -> Sum2/1
  init_condition_curr_point/1 -> Tl1/2
  from_prev_point/1 -> Gain19/1
  from_steam/1 -> Gain18/1

== system RC_top_ACU/Global Model RC/RC_top/C_liquide_3 ==
  from_steam : Inport
  from_prev_point : Inport  Port=2
  init_condition_curr_point : Inport  Port=3
  Gain18 : Gain  Gain=0.000006
  Gain19 : Gain  Gain=0.00004/1.17
  Gain22 : Gain  Gain=0.00004/1.17-(0.000006*0.000000000145)
  Sum2 : Sum  Inputs=-+-
  Tl1 : Integrator  InitialConditionSource=external  InitialCondition=124.3766
  to_steam : Outport
  to_next_point : Outport  Port=2
  wires:
  Gain22/1 -> Sum2/3
  Gain19/1 -> Sum2/2
  Sum2/1 -> Tl1/1
  Tl1/1 -> Gain22/1, to_steam/1, to_next_point/1
  Gain18/1 -> Sum2/1
  init_condition_curr_point/1 -> Tl1/2
  from_prev_point/1 -> Gain19/1
  from_steam/1 -> Gain18/1

== system RC_top_ACU/Global Model RC/RC_top/C_steam_1 ==
  from_T_prev_point : Inport
  from_T_curr_point : Inport  Port=2
  init_condition_curr_point : Inport  Port=3
  from_prev_point : Inport  Port=4
  from_liquid : Inport  Port=5
  Gain29 : Gain  Gain=0.000000000145
  Sum3 : Sum  Inputs=-+-
  Tp1 : Integrator  InitialConditionSource=external  InitialCondition=156.9966
  k1 : Subsystem
  speed : Subsystem
  to_next_point : Outport
  to_liquid : Outport  Port=2
  wires:
  init_condition_curr_point/1 -> Tp1/2
  speed/1(Out1) -> Sum3/2
  Gain29/1 -> Sum3/3
  Sum3/1 -> Tp1/1
  from_liquid/1 -> Gain29/1
  k1/1(Out1) -> Sum3/1
  Tp1/1 -> k1/2(In2), to_next_point/1, to_liquid/1
  from_T_curr_point/1 -> k1/1(In1)
  from_T_prev_point/1 -> speed/2(In2)
  from_prev_point/1 -> speed/1(In1)

== system RC_top_ACU/Global Model RC/RC_top/C_steam_2 ==
  from_T_prev_point : Inport
  from_T_curr_point : Inport  Port=2
  init_condition_curr_point : Inport  Port=3
  from_prev_point : Inport  Port=4
  from_liquid : Inport  Port=5
  Gain29 : Gain  Gain=0.004302*10^(-9)
  Sum3 : Sum  Inputs=-+-
  Tp1 : Integrator  InitialConditionSource=external  InitialCondition=156.9966
  k1 : Subsystem
  speed : Subsystem
  to_next_point : Outport
  to_liquid : Outport  Port=2
  wires:
  init_condition_curr_point/1 -> Tp1/2
  speed/1(Out1) -> Sum3/2
  Gain29/1 -> Sum3/3
  Sum3/1 -> Tp1/1
  from_liquid/1 -> Gain29/1
  k1/1(Out1) -> Sum3/1
  Tp1/1 -> k1/2(In2), to_next_point/1, to_liquid/1
  from_T_curr_point/1 -> k1/1(In1)
  from_prev_point/1 -> speed/1(In1)
  from_T_prev_point/1 -> speed/2(In2)

== system RC_top_ACU/Global Model RC/RC_top/C_steam_3 ==
  from_T_prev_point : Inport
  from_T_curr_point : Inport  Port=2
  init_condition_curr_point : Inport  Port=3
  from_prev_point : Inport  Port=4
  from_liquid : Inport  Port=5
  Gain29 : Gain  Gain=0.004302*10^(-9)
  Sum3 : Sum  Inputs=-+-
  Tp1 : Integrator  InitialConditionSource=external  InitialCondition=156.9966
  k1 : Subsystem
  speed : Subsystem
  to_next_point : Outport
  to_liquid : Outport  Port=2
  wires:
  init_condition_curr_point/1 -> Tp1/2
  speed/1(Out1) -> Sum3/2
  Gain29/1 -> Sum3/3
  Sum3/1 -> Tp1/1
  from_liquid/1 -> Gain29/1
  k1/1(Out1) -> Sum3/1
  Tp1/1 -> k1/2(In2), to_next_point/1, to_liquid/1
  from_T_curr_point/1 -> k1/1(In1)
  from_prev_point/1 -> speed/1(In1)
  from_T_prev_point/1 -> speed/2(In2)

== system RC_top_ACU/Global Model RC/RC_top/T_liquide_1 ==
  from_steam : Inport
  from_prev_point : Inport  Port=2
  init_condition_curr_point : Inport  Port=3
  Gain4 : Gain  Gain=0.0000855
  Gain5 : Gain  Gain=0.00004/1.17
  Gain8 : Gain  Gain=0.00004/1.17+0.0000855
  Sum2 : Sum  Inputs=++-
  Tl1 : Integrator  InitialConditionSource=external  InitialCondition=124.3766
  to_steam : Outport
  to_next_point : Outport  Port=2
  wires:
  Gain8/1 -> Sum2/3
  Gain5/1 -> Sum2/2
  Sum2/1 -> Tl1/1
  Tl1/1 -> to_steam/1, Gain8/1, to_next_point/1
  Gain4/1 -> Sum2/1
  init_condition_curr_point/1 -> Tl1/2
  from_prev_point/1 -> Gain5/1
  from_steam/1 -> Gain4/1

== system RC_top_ACU/Global Model RC/RC_top/T_liquide_2 ==
  from_steam : Inport
  from_prev_point : Inport  Port=2
  init_condition_curr_point : Inport  Port=3
  Gain4 : Gain  Gain=0.0000855
  Gain5 : Gain  Gain=0.00004/1.17
  Gain8 : Gain  Gain=0.00004/1.17+0.0000855
  Sum2 : Sum  Inputs=++-
  Tl1 : Integrator  InitialConditionSource=external  InitialCondition=124.3766
  to_steam : Outport
  to_next_point : Outport  Port=2
  wires:
  Gain8/1 -> Sum2/3
  Gain5/1 -> Sum2/2
  Sum2/1 -> Tl1/1
  Tl1/1 -> to_steam/1, Gain8/1, to_next_point/1
  Gain4/1 -> Sum2/1
  init_condition_curr_point/1 -> Tl1/2
  from_prev_point/1 -> Gain5/1
  from_steam/1 -> Gain4/1

== system RC_top_ACU/Global Model RC/RC_top/T_liquide_3 ==
  from_steam : Inport
  from_prev_point : Inport  Port=2
  init_condition_curr_point : Inport  Port=3
  Gain4 : Gain  Gain=0.0000855
  Gain5 : Gain  Gain=0.00004/1.17
  Gain8 : Gain  Gain=0.00004/1.17+0.0000855
  Sum2 : Sum  Inputs=++-
  Tl1 : Integrator  InitialConditionSource=external  InitialCondition=124.3766
  to_steam : Outport
  to_next_point : Outport  Port=2
  wires:
  Gain8/1 -> Sum2/3
  Gain5/1 -> Sum2/2
  Sum2/1 -> Tl1/1
  Tl1/1 -> to_steam/1, Gain8/1, to_next_point/1
  Gain4/1 -> Sum2/1
  init_condition_curr_point/1 -> Tl1/2
  from_prev_point/1 -> Gain5/1
  from_steam/1 -> Gain4/1

== system RC_top_ACU/Global Model RC/RC_top/T_steam_1 ==
  init_condition_curr_point : Inport
  from_prev_point : Inport  Port=2
  from_liquid : Inport  Port=3
  Gain33 : Gain  Gain=2.5
  Sum3 : Sum  Inputs=-++
  Tp : Integrator  InitialConditionSource=external  InitialCondition=156.9966
  k4 : Fcn  Expr=((0.002702752*(273.15+u))/1.17+2.5)*u
  speed3 : Fcn  Expr=(0.002702752*(273.15+u))/1.17*u
  to_concentration : Outport
  to_next_point : Outport  Port=2
  to_liquid : Outport  Port=3
  wires:
  init_condition_curr_point/1 -> Tp/2
  speed3/1 -> Sum3/2
  Gain33/1 -> Sum3/3
  Sum3/1 -> Tp/1
  from_prev_point/1 -> speed3/1
  k4/1 -> Sum3/1
  from_liquid/1 -> Gain33/1
  Tp/1 -> k4/1, to_concentration/1, to_next_point/1, to_liquid/1

== system RC_top_ACU/Global Model RC/RC_top/T_steam_2 ==
  init_condition_curr_point : Inport
  from_prev_point : Inport  Port=2
  from_liquid : Inport  Port=3
  Gain33 : Gain  Gain=2.5
  Sum3 : Sum  Inputs=-++
  Tp : Integrator  InitialConditionSource=external  InitialCondition=156.9966
  k4 : Fcn  Expr=((0.002702752*(273.15+u))/1.17+2.5)*u
  speed3 : Fcn  Expr=(0.002702752*(273.15+u))/1.17*u
  to_concentration : Outport
  to_next_point : Outport  Port=2
  to_liquid : Outport  Port=3
  wires:
  init_condition_curr_point/1 -> Tp/2
  speed3/1 -> Sum3/2
  Gain33/1 -> Sum3/3
  Sum3/1 -> Tp/1
  from_prev_point/1 -> speed3/1
  k4/1 -> Sum3/1
  from_liquid/1 -> Gain33/1
  Tp/1 -> k4/1, to_concentration/1, to_next_point/1, to_liquid/1

== system RC_top_ACU/Global Model RC/RC_top/T_steam_3 ==
  init_condition_curr_point : Inport
  from_prev_point : Inport  Port=2
  from_liquid : Inport  Port=3
  Gain33 : Gain  Gain=2.5
  Sum3 : Sum  Inputs=-++
  Tp : Integrator  InitialConditionSource=external  InitialCondition=156.9966
  k4 : Fcn  Expr=((0.002702752*(273.15+u))/1.17+2.5)*u
  speed3 : Fcn  Expr=(0.002702752*(273.15+u))/1.17*u
  to_concentration : Outport
  to_next_point : Outport  Port=2
  to_liquid : Outport  Port=3
  wires:
  init_condition_curr_point/1 -> Tp/2
  speed3/1 -> Sum3/2
  Gain33/1 -> Sum3/3
  Sum3/1 -> Tp/1
  from_prev_point/1 -> speed3/1
  k4/1 -> Sum3/1
  from_liquid/1 -> Gain33/1
  Tp/1 -> k4/1, to_concentration/1, to_next_point/1, to_liquid/1

== system RC_top_ACU/Global Model RC/RC_top/k1 ==
  In1 : Inport
  In2 : Inport  Port=2
  Product13 : Product  SaturateOnIntegerOverflow=on  InputSameDT=on  OutDataTypeStr=Inherit: Same as first input
  speed3 : Fcn  Expr=(0.002702752*(273.15+u))/1.17-0.147
  Out1 : Outport
  wires:
  Product13/1 -> Out1/1
  speed3/1 -> Product13/2
  In2/1 -> speed3/1
  In1/1 -> Product13/1

== system RC_top_ACU/Global Model RC/RC_top/k2 ==
  In1 : Inport
  In2 : Inport  Port=2
  Product13 : Product  SaturateOnIntegerOverflow=on  InputSameDT=on  OutDataTypeStr=Inherit: Same as first input
  speed3 : Fcn  Expr=(0.002702752*(273.15+u))/1.17-0.147
  Out1 : Outport
  wires:
  In1/1 -> Product13/1
  In2/1 -> speed3/1
  speed3/1 -> Product13/2
  Product13/1 -> Out1/1

== system RC_top_ACU/Global Model RC/RC_top/speed1 ==
  In1 : Inport
  In2 : Inport  Port=2
  Product13 : Product  SaturateOnIntegerOverflow=on  InputSameDT=on  OutDataTypeStr=Inherit: Same as first input
  speed3 : Fcn  Expr=(0.002702752*(273.15+u))/1.17
  Out1 : Outport
  wires:
  Product13/1 -> Out1/1
  speed3/1 -> Product13/2
  In2/1 -> speed3/1
  In1/1 -> Product13/1

== system RC_top_ACU/Global Model RC/RC_top/speed6 ==
  In1 : Inport
  In2 : Inport  Port=2
  Product13 : Product  SaturateOnIntegerOverflow=on  InputSameDT=on  OutDataTypeStr=Inherit: Same as first input
  speed3 : Fcn  Expr=(0.002702752*(273.15+u))/1.17
  Out1 : Outport
  wires:
  In1/1 -> Product13/1
  In2/1 -> speed3/1
  speed3/1 -> Product13/2
  Product13/1 -> Out1/1

== system RC_top_ACU/Global Model RC/ACU/ACU_1 /Pr.f ==
  In1 : Inport
  1/T : Gain
  Fcn : Fcn  Expr=(u/0.152)^(1/2)
  Gain1 : Gain
  "Gf, kmol/h1" : Display
  "Gf, kmol/h2" : Display
  Integrator : Integrator  InitialCondition=403.6
  Sum1 : Sum
  Sum2 : Sum  Inputs=-+
  Tst-t : Scope  NumInputPorts=3
  U1 : Constant  Value=380
  kn : Gain  Gain=4300
  Out1 : Outport
  wires:
  kn/1 -> 1/T/1, Gain1/1
  1/T/1 -> Integrator/1, "Gf, kmol/h1"/1
  Integrator/1 -> Sum1/2, Tst-t/3, "Gf, kmol/h2"/1
  Gain1/1 -> Sum1/1
  Sum1/1 -> Sum2/2
  U1/1 -> Sum2/1
  In1/1 -> kn/1
  Fcn/1 -> Tst-t/1, Out1/1
  Sum2/1 -> Tst-t/2, Fcn/1

== system RC_top_ACU/Global Model RC/ACU/ACU_1 /SbS RASCHET G ==
  In1 : Inport
  In2 : Inport  Port=2
  In3 : Inport  Port=3
  In4 : Inport  Port=4
  "Cd, mol.dol" : Fcn  Expr=(u/18.02)/((u/18.02)+((1-u)/106.12))
  "Cna, mol.dol" : Fcn  Expr=(u/18.02)/((u/18.02)+((1-u)/106.12))
  "Cra, mol.dol" : Fcn  Expr=(u/18.02)/((u/18.02)+((1-u)/106.12))
  Fcn1 : Fcn  Expr=1/u
  Fcn10 : Fcn  Expr=1/u
  Fcn6 : Fcn  Expr=1/u
  Gd*(R+1) : Fcn  Expr=u*(0.5+1)
  Gd*R : Fcn  Expr=u*0.5
  "Md, kg/kmol" : Fcn  Expr=18.02*u+106.12*(1-u)
  "Mna, kg/kmol1" : Fcn  Expr=18.02*u+106.12*(1-u)
  "Mra, kg/kmol" : Fcn  Expr=18.02*u+106.12*(1-u)
  Pr{,1..8} (9 alike) : Product  RndMeth=Zero
  Sbtr2 : Sum  Inputs=+-
  Sbtr3 : Sum  Inputs=-+
  Str : Sum  Inputs=-+
  Str1 : Sum  Inputs=-+
  Out1 : Outport
  Out2 : Outport  Port=2
  Out3 : Outport  Port=3
  Out4 : Outport  Port=4
  Out5 : Outport  Port=5
  Out6 : Outport  Port=6
  Out7 : Outport  Port=7
  Out8 : Outport  Port=8
  Out9 : Outport  Port=9
  wires:
  "Mna, kg/kmol1"/1 -> Pr3/1
  "Cna, mol.dol"/1 -> "Mna, kg/kmol1"/1, Str/1, Sbtr3/1, Sbtr2/1
  "Cra, mol.dol"/1 -> "Mra, kg/kmol"/1, Str1/1, Sbtr3/2
  "Cd, mol.dol"/1 -> "Md, kg/kmol"/1, Str1/2, Str/2, Sbtr2/2
  "Mra, kg/kmol"/1 -> Fcn6/1
  Fcn6/1 -> Pr/2
  Pr/1 -> Pr2/1, Out3/1, Pr5/1
  Str/1 -> Fcn10/1
  Fcn10/1 -> Pr1/2
  Pr2/1 -> Pr3/2, Out2/1
  Pr1/1 -> Pr2/2
  Str1/1 -> Pr1/1
  Fcn1/1 -> Pr4/2
  Pr5/1 -> Pr6/1, Gd*(R+1)/1, Gd*R/1, Out4/1
  Pr4/1 -> Pr5/2
  "Md, kg/kmol"/1 -> Pr6/2, Pr7/2, Pr8/2
  Sbtr2/1 -> Fcn1/1
  Sbtr3/1 -> Pr4/1
  Gd*(R+1)/1 -> Pr7/1, Out6/1
  Gd*R/1 -> Pr8/1, Out8/1
  In1/1 -> "Cna, mol.dol"/1
  Pr3/1 -> Out1/1
  In2/1 -> Pr/1
  In3/1 -> "Cra, mol.dol"/1
  Pr6/1 -> Out5/1
  In4/1 -> "Cd, mol.dol"/1
  Pr7/1 -> Out7/1
  Pr8/1 -> Out9/1

== system RC_top_ACU/Global Model RC/ACU/C_steam_1/k1 ==
  In1 : Inport
  In2 : Inport  Port=2
  EVAP_params1 : Inport  Port=3
  Coeff : Constant  Value=0.785
  Demux : Demux  Outputs=6
  Display : Display
  Display1 : Display
  Display2 : Display
  Divide : Product  Inputs=*/
  Divide1 : Product  Inputs=*/
  Product1 : Product  Inputs=4  SaturateOnIntegerOverflow=on  InputSameDT=on  OutDataTypeStr=Inherit: Same as first input
  Product13 : Product  SaturateOnIntegerOverflow=on  InputSameDT=on  OutDataTypeStr=Inherit: Same as first input
  Product2 : Product  Inputs=4  SaturateOnIntegerOverflow=on  InputSameDT=on  OutDataTypeStr=Inherit: Same as first input
  Product3 : Product  SaturateOnIntegerOverflow=on  InputSameDT=on  OutDataTypeStr=Inherit: Same as first input
  Product4 : Product  SaturateOnIntegerOverflow=on  InputSameDT=on  OutDataTypeStr=Inherit: Same as first input
  Sum : Sum  Inputs=++|
  Sum1 : Sum  Inputs=|+-
  T_0 : Constant  Value=273.15
  T_1 : Constant  Value=273.15
  T_2 : Constant  Value=0.0000216487318
  T_3 : Constant  Value=0.003223135
  speed3 : Fcn  Expr=((0.003223135*(273+u))/24.69822264)/1.375-0.004302
  Out1 : Outport
  wires:
  speed3/1 -> Product13/1
  T_1/1 -> Product2/4
  Divide/1 -> Divide1/1
  EVAP_params1/1 -> Demux/1
  Demux/1 -> Divide1/2
  Demux/6 -> Product4/2, Product4/1
  In2/1 -> Product3/1, Product13/2
  Coeff/1 -> Product2/3
  In1/1 -> Sum/1, speed3/1
  Demux/4 -> Product1/4
  Demux/5 -> Product2/1
  Demux/3 -> Product1/3
  Product4/1 -> Product2/2
  Product3/1 -> Out1/1, Display/1
  T_0/1 -> Sum/2
  Product1/1 -> Divide/1
  Sum/1 -> Product1/1
  Demux/2 -> Product1/2
  Product13/1 -> Display1/1
  Sum1/1 -> Product3/2
  Divide1/1 -> Sum1/1
  T_2/1 -> Sum1/2
  T_3/1 -> Display2/1
  Product2/1 -> Divide/2
